simulink model "bio_matfunc_quat_error"  (R2017b)
settings: Solver=VariableStepAuto  StartTime=0.0  StopTime=10.0  RelTol=1e-3
settings Model: Creator=ktrinh  LastModifiedBy=ktrinh

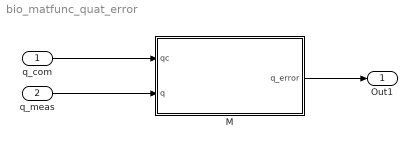
== system bio_matfunc_quat_error ==
  q_com : Inport  OutDataTypeStr=double  PortDimensions=4
  q_meas : Inport  Port=2  OutDataTypeStr=double  PortDimensions=4
  M : MATLAB Function  TreatAsAtomicUnit=on
  Out1 : Outport
  wires:
  q_com/1 -> M/1(qc)
  q_meas/1 -> M/2(q)
  M/1(q_error) -> Out1/1

== matlab function bio_matfunc_quat_error/M ==
  data: qc input; q input; q_error output
function q_error = quat_error(qc,q)
%#codegen

%qc = q_comm
%q = q_meas

qcm = [qc(4) qc(3) -qc(2) -qc(1);
       -qc(3) qc(4) qc(1) -qc(2);
       qc(2) -qc(1) qc(4) -qc(3);
       qc(1) qc(2) qc(3) qc(4)];

q_error = qcm*[q(1);q(2);q(3);q(4)];
